simulink model "Lcontainer_simNN"  (R2018b)
settings: Solver=FixedStepAuto  StartTime=0.0  StopTime=600  FixedStep=0.1  RelTol=1e-3
libraries: neural x88, simulink x1
(part 2 of 4)

== system Lcontainer_simNN/LContainer Controller/Layer 2/Delays 1 ==
  "p{2}" : Inport  PortDimensions=10
      mask Display: e = 0.06;c1 = [120 230 180]/255;c2 = ([120 230 180]+0)/(256+128);c3 = ([120 230 180]+128)/(256+128);patch([0 1 1 0],[0 0 1 1],c1);patch([0 1 1 1-e 1-e 0+e],[0 0 1 1-e 0+e 0+e],c2);patch([0 0 1 1-e 0+e 0+e],[0 1 1 1-e 1-e 0+e],c3);plot([0 1 1 0 0],[0 0 1 1 0]);
  mux : Mux  Inputs=1
      mask Display: e = 0.06;c1 = [120 150 230]/255;c2 = ([120 150 230]+0)/383;c3 = ([120 150 230]+128)/383;patch([0 1 1 0],[0 0 1 1],c1);patch([0 1 1 1-e 1-e 0+e],[0 0 1 1-e 0+e 0+e],c2);patch([0 0 1 1-e 0+e 0+e],[0 1 1 1-e 1-e 0+e],c3);plot([0 1 1 0 0],[0 0 1 1 0]);disp('Mux')
  "pd{2,1}" : Outport
      mask Display: e = 0.06;c1 = [120 230 180]/255;c2 = ([120 230 180]+0)/(256+128);c3 = ([120 230 180]+128)/(256+128);patch([0 1 1 0],[0 0 1 1],c1);patch([0 1 1 1-e 1-e 0+e],[0 0 1 1-e 0+e 0+e],c2);patch([0 0 1 1-e 0+e 0+e],[0 1 1 1-e 1-e 0+e],c3);plot([0 1 1 0 0],[0 0 1 1 0]);
  wires:
  mux/1 -> "pd{2,1}"/1
  "p{2}"/1 -> mux/1

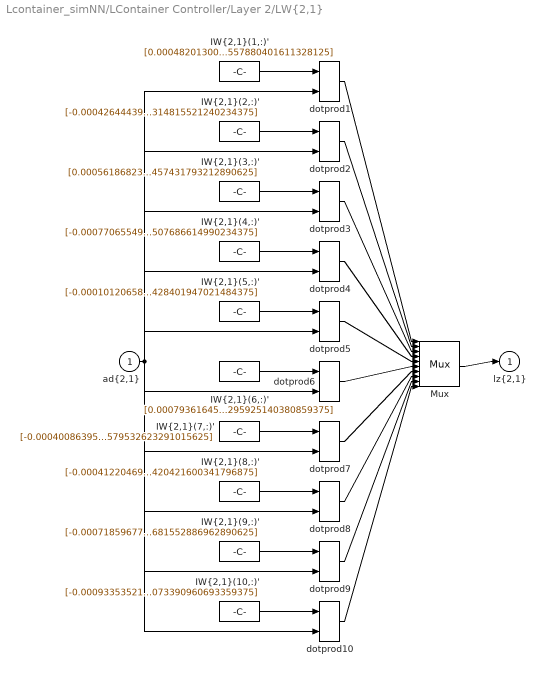
== system Lcontainer_simNN/LContainer Controller/Layer 2/LW{2,1} ==
  "ad{2,1}" : Inport  PortDimensions=10
      mask Display: e = 0.06;c1 = [120 230 180]/255;c2 = ([120 230 180]+0)/(256+128);c3 = ([120 230 180]+128)/(256+128);patch([0 1 1 0],[0 0 1 1],c1);patch([0 1 1 1-e 1-e 0+e],[0 0 1 1-e 0+e 0+e],c2);patch([0 0 1 1-e 0+e 0+e],[0 1 1 1-e 1-e 0+e],c3);plot([0 1 1 0 0],[0 0 1 1 0]);
  "IW{2,1}(1,:)'" : Constant  Value=[0.0004820130050322240893023728602884148131124675273895263671875;-0.14897274999759291258527582613169215619564056396484375;0.0087908951607520609272672373890600283630192279815673828125;-0.053122726519414069368263398018825682811439037322998046875;0.0002402089536153212585845029281017559696920216083526611328125;0.00659270133509061440069132231656112708151340484619140625;0.047066903764155669509516854986941325478255748748779296875;-0.00070479248297768896762416357404390510055236518383026123046875;-0.0302802175473580355291591814648199942894279956817626953125;0.0166965879907191756814643923689800431020557880401611328125]
      mask Display: e = 0.06;c1 = [120 150 230]/255;c2 = ([120 150 230]+0)/383;c3 = ([120 150 230]+128)/383;patch([0 1 1 0],[0 0 1 1],c1);patch([0 1 1 1-e 1-e 0+e],[0 0 1 1-e 0+e 0+e],c2);patch([0 0 1 1-e 0+e 0+e],[0 1 1 1-e 1-e 0+e],c3);plot([0 1 1 0 0],[0 0 1 1 0]);disp('weights');
  "IW{2,1}(10,:)'" : Constant  Value=[-0.000933535212733850269274660238494334407732822000980377197265625;-0.000772387208203969177940095836021328068454749882221221923828125;0.000783528929132344871023863053238756037899293005466461181640625;0.000744496740820047540887482995231039240024983882904052734375;-0.000748280223311167231280138789628608719795010983943939208984375;-0.000336708204216668006113211131236084838747046887874603271484375;-0.000636414158899125162981158521091629154398106038570404052734375;-0.000932538469281236057951967044488128522061742842197418212890625;0.000166570528255750231576282072154526758822612464427947998046875;0.0001092356001364544275909762571785677209845744073390960693359375]
      mask Display: e = 0.06;c1 = [120 150 230]/255;c2 = ([120 150 230]+0)/383;c3 = ([120 150 230]+128)/383;patch([0 1 1 0],[0 0 1 1],c1);patch([0 1 1 1-e 1-e 0+e],[0 0 1 1-e 0+e 0+e],c2);patch([0 0 1 1-e 0+e 0+e],[0 1 1 1-e 1-e 0+e],c3);plot([0 1 1 0 0],[0 0 1 1 0]);disp('weights');
  "IW{2,1}(2,:)'" : Constant  Value=[-0.0004264443902295060964159623129177134615019895136356353759765625;-0.000560105703268952924943346882713512968621216714382171630859375;0.000377584095749465358492213962193773113540373742580413818359375;-0.000700634792845798346459795791218994054361246526241302490234375;0.0004874063537030847402531374967793453834019601345062255859375;-9.7285835613794088990412267659024792010313831269741058349609375e-05;0.000749616668439126465108002239645657027722336351871490478515625;0.00084023165745046525694494921054911173996515572071075439453125;-0.000916171932540294788570311990127947865403257310390472412109375;0.000118539205010998924781639995984505731030367314815521240234375]
      mask Display: e = 0.06;c1 = [120 150 230]/255;c2 = ([120 150 230]+0)/383;c3 = ([120 150 230]+128)/383;patch([0 1 1 0],[0 0 1 1],c1);patch([0 1 1 1-e 1-e 0+e],[0 0 1 1-e 0+e 0+e],c2);patch([0 0 1 1-e 0+e 0+e],[0 1 1 1-e 1-e 0+e],c3);plot([0 1 1 0 0],[0 0 1 1 0]);disp('weights');
  "IW{2,1}(3,:)'" : Constant  Value=[0.000561868235751858554304083437358485753065906465053558349609375;-0.0004553795308148002145276489471825698274187743663787841796875;-0.00016668990031184395951384391576510779486852698028087615966796875;0.000597047158527498384068821213332967090536840260028839111328125;-0.0002934852706778429457488976961343496441259048879146575927734375;0.00015225641794986368338267468391933334714849479496479034423828125;-0.0002772254366225171428629592274006654406548477709293365478515625;0.0003822805927828255173096805297205946772010065615177154541015625;-0.000492935117287975348328299407540953325224108994007110595703125;-0.000934933027334356446004515195369322100304998457431793212890625]
      mask Display: e = 0.06;c1 = [120 150 230]/255;c2 = ([120 150 230]+0)/383;c3 = ([120 150 230]+128)/383;patch([0 1 1 0],[0 0 1 1],c1);patch([0 1 1 1-e 1-e 0+e],[0 0 1 1-e 0+e 0+e],c2);patch([0 0 1 1-e 0+e 0+e],[0 1 1 1-e 1-e 0+e],c3);plot([0 1 1 0 0],[0 0 1 1 0]);disp('weights');
  "IW{2,1}(4,:)'" : Constant  Value=[-0.0007706554936704437981653814659921408747322857379913330078125;0.005736968078448979359296178159866030910052359104156494140625;-0.0215993275616708467479210042938575497828423976898193359375;0.0275851081881576011556322924889173009432852268218994140625;-0.0004468698480519939383003025223928261766559444367885589599609375;-0.0032100621946929267826187359702316825860179960727691650390625;-0.0148528526677068895001099235742003656923770904541015625;-0.00084295935895107947620485955297908731154166162014007568359375;0.0162611889792566959023201178524686838500201702117919921875;-0.03252290811202539211333117918911739252507686614990234375]
      mask Display: e = 0.06;c1 = [120 150 230]/255;c2 = ([120 150 230]+0)/383;c3 = ([120 150 230]+128)/383;patch([0 1 1 0],[0 0 1 1],c1);patch([0 1 1 1-e 1-e 0+e],[0 0 1 1-e 0+e 0+e],c2);patch([0 0 1 1-e 0+e 0+e],[0 1 1 1-e 1-e 0+e],c3);plot([0 1 1 0 0],[0 0 1 1 0]);disp('weights');
  "IW{2,1}(5,:)'" : Constant  Value=[-0.000101206583531268193309506087107507710243226028978824615478515625;-0.000867505466564442322997818823893112494261004030704498291015625;6.972171281489726916112681376347381956293247640132904052734375e-05;-0.0006499836952546214803583257690888785873539745807647705078125;0.000768931164791470550014251816861587940366007387638092041015625;-0.00051077340179170381377626863894647613051347434520721435546875;0.0002396027776789714049988921917844209019676782190799713134765625;0.0004961867667277962933025658998076323769055306911468505859375;7.5421709981156692215002734780426862926105968654155731201171875e-05;-0.0005186449873913457318808095664053325890563428401947021484375]
      mask Display: e = 0.06;c1 = [120 150 230]/255;c2 = ([120 150 230]+0)/383;c3 = ([120 150 230]+128)/383;patch([0 1 1 0],[0 0 1 1],c1);patch([0 1 1 1-e 1-e 0+e],[0 0 1 1-e 0+e 0+e],c2);patch([0 0 1 1-e 0+e 0+e],[0 1 1 1-e 1-e 0+e],c3);plot([0 1 1 0 0],[0 0 1 1 0]);disp('weights');
  "IW{2,1}(6,:)'" : Constant  Value=[0.000793616452609966350865977613437962645548395812511444091796875;0.0072189631106161604445770052507214131765067577362060546875;-0.025168099441065662491556764734923490323126316070556640625;0.03499676826161253473390644330720533616840839385986328125;-0.00013966872952280381145299947842630672312225215137004852294921875;-0.002944584517023267171420553012239906820468604564666748046875;-0.0201810876198396278724533914328276296146214008331298828125;0.000493104595042109512641193003190664967405609786510467529296875;0.0192394162008955559028944293231688789092004299163818359375;-0.040115708372885826304976575329419574700295925140380859375]
      mask Display: e = 0.06;c1 = [120 150 230]/255;c2 = ([120 150 230]+0)/383;c3 = ([120 150 230]+128)/383;patch([0 1 1 0],[0 0 1 1],c1);patch([0 1 1 1-e 1-e 0+e],[0 0 1 1-e 0+e 0+e],c2);patch([0 0 1 1-e 0+e 0+e],[0 1 1 1-e 1-e 0+e],c3);plot([0 1 1 0 0],[0 0 1 1 0]);disp('weights');
  "IW{2,1}(7,:)'" : Constant  Value=[-0.000400863950280058961399276551418324743281118571758270263671875;-0.0225465071540020926821323854483125614933669567108154296875;-0.0280520076515327794475229694626250420697033405303955078125;-0.00942244816999010005587056326703532249666750431060791015625;0.000902860424200245472066417296019835703191347420215606689453125;0.001138975060225336406738438910224431310780346393585205078125;-0.041810146757115640436808234881027601659297943115234375;0.000821642012028902537189301025222221142030321061611175537109375;-0.004447628372272441517332186577959873829968273639678955078125;-0.0285545253020185775538752892543925554491579532623291015625]
      mask Display: e = 0.06;c1 = [120 150 230]/255;c2 = ([120 150 230]+0)/383;c3 = ([120 150 230]+128)/383;patch([0 1 1 0],[0 0 1 1],c1);patch([0 1 1 1-e 1-e 0+e],[0 0 1 1-e 0+e 0+e],c2);patch([0 0 1 1-e 0+e 0+e],[0 1 1 1-e 1-e 0+e],c3);plot([0 1 1 0 0],[0 0 1 1 0]);disp('weights');
  "IW{2,1}(8,:)'" : Constant  Value=[-0.0004122046906352632247329259573831450325087644159793853759765625;-0.50634105157552655729347179658361710608005523681640625;-1.8097291749770356705795393281732685863971710205078125;-0.05223922011666985720790279401626321487128734588623046875;0.000317452984005011664379869440466563901281915605068206787109375;0.00478766364779581975186228959273648797534406185150146484375;-1.1621848213912837621819562627933919429779052734375;0.0004108452670455737111392113813934656718629412353038787841796875;-0.0302623349342728935329471795512290555052459239959716796875;-0.2779400021529727649038932213443331420421600341796875]
      mask Display: e = 0.06;c1 = [120 150 230]/255;c2 = ([120 150 230]+0)/383;c3 = ([120 150 230]+128)/383;patch([0 1 1 0],[0 0 1 1],c1);patch([0 1 1 1-e 1-e 0+e],[0 0 1 1-e 0+e 0+e],c2);patch([0 0 1 1-e 0+e 0+e],[0 1 1 1-e 1-e 0+e],c3);plot([0 1 1 0 0],[0 0 1 1 0]);disp('weights');
  "IW{2,1}(9,:)'" : Constant  Value=[-0.000718596778329273484613171074641968516516499221324920654296875;0.1351387556832968350750689978667651303112506866455078125;-0.069675559698190669966066934648551978170871734619140625;-0.038467952192683417533825007694758824072778224945068359375;0.00023637001640757784003132879746544858790002763271331787109375;0.004472859878445143051728383198906158213503658771514892578125;0.0194364277021570053261001476130331866443157196044921875;-0.00072977980434176729744588651982439841958694159984588623046875;-0.0222208908663231972935303559779640636406838893890380859375;-0.424243744226951324804986143135465681552886962890625]
      mask Display: e = 0.06;c1 = [120 150 230]/255;c2 = ([120 150 230]+0)/383;c3 = ([120 150 230]+128)/383;patch([0 1 1 0],[0 0 1 1],c1);patch([0 1 1 1-e 1-e 0+e],[0 0 1 1-e 0+e 0+e],c2);patch([0 0 1 1-e 0+e 0+e],[0 1 1 1-e 1-e 0+e],c3);plot([0 1 1 0 0],[0 0 1 1 0]);disp('weights');
  Mux : Mux  Inputs=10
      mask Display: e = 0.06;c1 = [120 150 230]/255;c2 = ([120 150 230]+0)/383;c3 = ([120 150 230]+128)/383;patch([0 1 1 0],[0 0 1 1],c1);patch([0 1 1 1-e 1-e 0+e],[0 0 1 1-e 0+e 0+e],c2);patch([0 0 1 1-e 0+e 0+e],[0 1 1 1-e 1-e 0+e],c3);plot([0 1 1 0 0],[0 0 1 1 0]);disp('Mux');
  dotprod{1..10} (10 alike) : neural/Weight Functions/dotprod
  "lz{2,1}" : Outport
      mask Display: e = 0.06;c1 = [120 230 180]/255;c2 = ([120 230 180]+0)/(256+128);c3 = ([120 230 180]+128)/(256+128);patch([0 1 1 0],[0 0 1 1],c1);patch([0 1 1 1-e 1-e 0+e],[0 0 1 1-e 0+e 0+e],c2);patch([0 0 1 1-e 0+e 0+e],[0 1 1 1-e 1-e 0+e],c3);plot([0 1 1 0 0],[0 0 1 1 0]);
  wires:
  Mux/1 -> "lz{2,1}"/1
  dotprod10/1 -> Mux/10
  "IW{2,1}(10,:)'"/1 -> dotprod10/1
  dotprod9/1 -> Mux/9
  "IW{2,1}(9,:)'"/1 -> dotprod9/1
  dotprod8/1 -> Mux/8
  "IW{2,1}(8,:)'"/1 -> dotprod8/1
  dotprod7/1 -> Mux/7
  "IW{2,1}(7,:)'"/1 -> dotprod7/1
  dotprod6/1 -> Mux/6
  "IW{2,1}(6,:)'"/1 -> dotprod6/1
  dotprod5/1 -> Mux/5
  "IW{2,1}(5,:)'"/1 -> dotprod5/1
  dotprod4/1 -> Mux/4
  "IW{2,1}(4,:)'"/1 -> dotprod4/1
  dotprod3/1 -> Mux/3
  "IW{2,1}(3,:)'"/1 -> dotprod3/1
  dotprod2/1 -> Mux/2
  "IW{2,1}(2,:)'"/1 -> dotprod2/1
  dotprod1/1 -> Mux/1
  "ad{2,1}"/1 -> dotprod10/2, dotprod9/2, dotprod8/2, dotprod7/2, dotprod6/2, dotprod5/2, dotprod4/2, dotprod3/2, dotprod2/2, dotprod1/2
  "IW{2,1}(1,:)'"/1 -> dotprod1/1

== system Lcontainer_simNN/LContainer Controller/Layer 3/Delays 1 ==
  "p{3}" : Inport  PortDimensions=10
      mask Display: e = 0.06;c1 = [120 230 180]/255;c2 = ([120 230 180]+0)/(256+128);c3 = ([120 230 180]+128)/(256+128);patch([0 1 1 0],[0 0 1 1],c1);patch([0 1 1 1-e 1-e 0+e],[0 0 1 1-e 0+e 0+e],c2);patch([0 0 1 1-e 0+e 0+e],[0 1 1 1-e 1-e 0+e],c3);plot([0 1 1 0 0],[0 0 1 1 0]);
  mux : Mux  Inputs=1
      mask Display: e = 0.06;c1 = [120 150 230]/255;c2 = ([120 150 230]+0)/383;c3 = ([120 150 230]+128)/383;patch([0 1 1 0],[0 0 1 1],c1);patch([0 1 1 1-e 1-e 0+e],[0 0 1 1-e 0+e 0+e],c2);patch([0 0 1 1-e 0+e 0+e],[0 1 1 1-e 1-e 0+e],c3);plot([0 1 1 0 0],[0 0 1 1 0]);disp('Mux')
  "pd{3,2}" : Outport
      mask Display: e = 0.06;c1 = [120 230 180]/255;c2 = ([120 230 180]+0)/(256+128);c3 = ([120 230 180]+128)/(256+128);patch([0 1 1 0],[0 0 1 1],c1);patch([0 1 1 1-e 1-e 0+e],[0 0 1 1-e 0+e 0+e],c2);patch([0 0 1 1-e 0+e 0+e],[0 1 1 1-e 1-e 0+e],c3);plot([0 1 1 0 0],[0 0 1 1 0]);
  wires:
  mux/1 -> "pd{3,2}"/1
  "p{3}"/1 -> mux/1

== system Lcontainer_simNN/LContainer Controller/Layer 3/LW{3,2} ==
  "ad{3,2}" : Inport  PortDimensions=10
      mask Display: e = 0.06;c1 = [120 230 180]/255;c2 = ([120 230 180]+0)/(256+128);c3 = ([120 230 180]+128)/(256+128);patch([0 1 1 0],[0 0 1 1],c1);patch([0 1 1 1-e 1-e 0+e],[0 0 1 1-e 0+e 0+e],c2);patch([0 0 1 1-e 0+e 0+e],[0 1 1 1-e 1-e 0+e],c3);plot([0 1 1 0 0],[0 0 1 1 0]);
  "IW{3,2}(1,:)'" : Constant  Value=[-0.272649380870168211998816332197748124599456787109375;0.00013227176168331794786463262436626564522157423198223114013671875;-0.00057629457199402677781974180248880657018162310123443603515625;-0.00594714213795307679311097359686755225993692874908447265625;0.0004735837959567169006859510549389824518584646284580230712890625;-0.037568305788482865559263501609166269190609455108642578125;0.00724237752689754592239079755700004170648753643035888671875;-2.15262859222610369869244095752947032451629638671875;0.058953518285207950899717843640246428549289703369140625;-0.00050529459321236648051967055295108366408385336399078369140625]
      mask Display: e = 0.06;c1 = [120 150 230]/255;c2 = ([120 150 230]+0)/383;c3 = ([120 150 230]+128)/383;patch([0 1 1 0],[0 0 1 1],c1);patch([0 1 1 1-e 1-e 0+e],[0 0 1 1-e 0+e 0+e],c2);patch([0 0 1 1-e 0+e 0+e],[0 1 1 1-e 1-e 0+e],c3);plot([0 1 1 0 0],[0 0 1 1 0]);disp('weights');
  Mux : Mux  Inputs=1
      mask Display: e = 0.06;c1 = [120 150 230]/255;c2 = ([120 150 230]+0)/383;c3 = ([120 150 230]+128)/383;patch([0 1 1 0],[0 0 1 1],c1);patch([0 1 1 1-e 1-e 0+e],[0 0 1 1-e 0+e 0+e],c2);patch([0 0 1 1-e 0+e 0+e],[0 1 1 1-e 1-e 0+e],c3);plot([0 1 1 0 0],[0 0 1 1 0]);disp('Mux');
  dotprod1 : neural/Weight Functions/dotprod
  "lz{3,2}" : Outport
      mask Display: e = 0.06;c1 = [120 230 180]/255;c2 = ([120 230 180]+0)/(256+128);c3 = ([120 230 180]+128)/(256+128);patch([0 1 1 0],[0 0 1 1],c1);patch([0 1 1 1-e 1-e 0+e],[0 0 1 1-e 0+e 0+e],c2);patch([0 0 1 1-e 0+e 0+e],[0 1 1 1-e 1-e 0+e],c3);plot([0 1 1 0 0],[0 0 1 1 0]);
  wires:
  Mux/1 -> "lz{3,2}"/1
  dotprod1/1 -> Mux/1
  "ad{3,2}"/1 -> dotprod1/2
  "IW{3,2}(1,:)'"/1 -> dotprod1/1

== system Lcontainer_simNN/LContainer Plant/Layer 1/Delays 1 ==
  "p{1}" : Inport  PortDimensions=10
      mask Display: e = 0.06;c1 = [120 230 180]/255;c2 = ([120 230 180]+0)/(256+128);c3 = ([120 230 180]+128)/(256+128);patch([0 1 1 0],[0 0 1 1],c1);patch([0 1 1 1-e 1-e 0+e],[0 0 1 1-e 0+e 0+e],c2);patch([0 0 1 1-e 0+e 0+e],[0 1 1 1-e 1-e 0+e],c3);plot([0 1 1 0 0],[0 0 1 1 0]);
  mux : Mux  Inputs=1
      mask Display: e = 0.06;c1 = [120 150 230]/255;c2 = ([120 150 230]+0)/383;c3 = ([120 150 230]+128)/383;patch([0 1 1 0],[0 0 1 1],c1);patch([0 1 1 1-e 1-e 0+e],[0 0 1 1-e 0+e 0+e],c2);patch([0 0 1 1-e 0+e 0+e],[0 1 1 1-e 1-e 0+e],c3);plot([0 1 1 0 0],[0 0 1 1 0]);disp('Mux')
  "pd{1,1}" : Outport
      mask Display: e = 0.06;c1 = [120 230 180]/255;c2 = ([120 230 180]+0)/(256+128);c3 = ([120 230 180]+128)/(256+128);patch([0 1 1 0],[0 0 1 1],c1);patch([0 1 1 1-e 1-e 0+e],[0 0 1 1-e 0+e 0+e],c2);patch([0 0 1 1-e 0+e 0+e],[0 1 1 1-e 1-e 0+e],c3);plot([0 1 1 0 0],[0 0 1 1 0]);
  wires:
  mux/1 -> "pd{1,1}"/1
  "p{1}"/1 -> mux/1

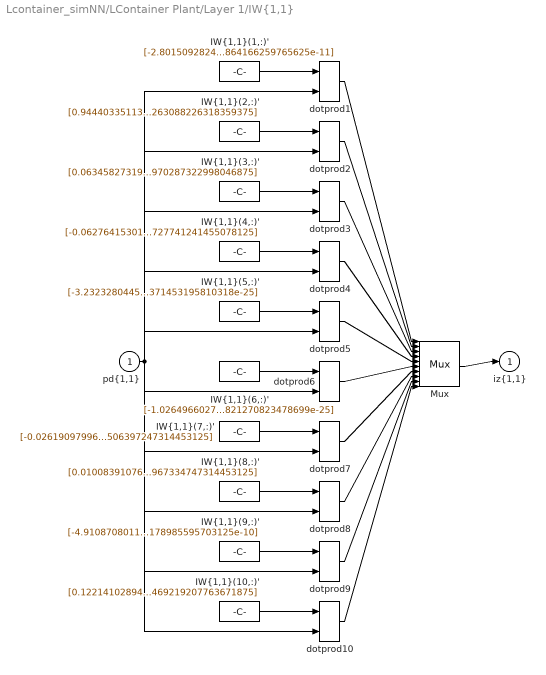
== system Lcontainer_simNN/LContainer Plant/Layer 1/IW{1,1} ==
  "pd{1,1}" : Inport  PortDimensions=10
      mask Display: e = 0.06;c1 = [120 230 180]/255;c2 = ([120 230 180]+0)/(256+128);c3 = ([120 230 180]+128)/(256+128);patch([0 1 1 0],[0 0 1 1],c1);patch([0 1 1 1-e 1-e 0+e],[0 0 1 1-e 0+e 0+e],c2);patch([0 0 1 1-e 0+e 0+e],[0 1 1 1-e 1-e 0+e],c3);plot([0 1 1 0 0],[0 0 1 1 0]);
  "IW{1,1}(1,:)'" : Constant  Value=[-2.801509282442014055289999211492517339205932103141094557940959930419921875e-09;6.48709663420110913726937300883526767159015236074992571957409381866455078125e-11;-1.38806045741189341650107961675240076889793761072411371060297824442386627197265625e-12;-6.949262728077942046686543068993724414639245878788642585277557373046875e-10;4.9583045758239326267706093454186444535736200123210437595844268798828125e-09;7.20807982755057124969425602884896237096575000169451641340856440365314483642578125e-13;1.47915336545584584323170595539991166640116093677903563730069436132907867431640625e-12;1.368467688852383455193129604555463631654528555703365100271184928715229034423828125e-13;-2.4782259643928960868026404257559685943845817490682748029939830303192138671875e-11;-2.17656041339324496223947102679151612870944720867782962159253656864166259765625e-11]
      mask Display: e = 0.06;c1 = [120 150 230]/255;c2 = ([120 150 230]+0)/383;c3 = ([120 150 230]+128)/383;patch([0 1 1 0],[0 0 1 1],c1);patch([0 1 1 1-e 1-e 0+e],[0 0 1 1-e 0+e 0+e],c2);patch([0 0 1 1-e 0+e 0+e],[0 1 1 1-e 1-e 0+e],c3);plot([0 1 1 0 0],[0 0 1 1 0]);disp('Weights');
  "IW{1,1}(10,:)'" : Constant  Value=[0.1221410289429804285621372628156677819788455963134765625;-0.06221579091204963718464426847276627086102962493896484375;0.00077577425811804832760099071009562976541928946971893310546875;0.0057878098276135346578197271583121619187295436859130859375;-0.29336456194867477353938056694460101425647735595703125;-0.00153674477675105609734973466373730843770317733287811279296875;-0.01024849367676159382634093475417103036306798458099365234375;0.07417790242423320801190556039728107862174510955810546875;-0.1474125279109223252138605175787233747541904449462890625;0.67016334654499143397288207779638469219207763671875]
      mask Display: e = 0.06;c1 = [120 150 230]/255;c2 = ([120 150 230]+0)/383;c3 = ([120 150 230]+128)/383;patch([0 1 1 0],[0 0 1 1],c1);patch([0 1 1 1-e 1-e 0+e],[0 0 1 1-e 0+e 0+e],c2);patch([0 0 1 1-e 0+e 0+e],[0 1 1 1-e 1-e 0+e],c3);plot([0 1 1 0 0],[0 0 1 1 0]);disp('Weights');
  "IW{1,1}(2,:)'" : Constant  Value=[0.94440335113838036473765669143176637589931488037109375;-0.1629366186686034001507294988186913542449474334716796875;0.0014086521436272440334358524438584936433471739292144775390625;0.0011875416120418805752956270538334138109348714351654052734375;-0.0095127288471239003497803565778667689301073551177978515625;-0.030355092939376430993814182102141785435378551483154296875;-0.027077648132769714661716164982863119803369045257568359375;-0.0214545100883952628845197097007257980294525623321533203125;0.0221409157462193577348141815264170872978866100311279296875;-0.0799528339554468059358072196118882857263088226318359375]
      mask Display: e = 0.06;c1 = [120 150 230]/255;c2 = ([120 150 230]+0)/383;c3 = ([120 150 230]+128)/383;patch([0 1 1 0],[0 0 1 1],c1);patch([0 1 1 1-e 1-e 0+e],[0 0 1 1-e 0+e 0+e],c2);patch([0 0 1 1-e 0+e 0+e],[0 1 1 1-e 1-e 0+e],c3);plot([0 1 1 0 0],[0 0 1 1 0]);disp('Weights');
  "IW{1,1}(3,:)'" : Constant  Value=[0.06345827319009154920959048240547417663037776947021484375;-0.002284892575671929569602891518798060133121907711029052734375;-3.8590476702913398461027016939084433033713139593601226806640625e-05;-0.0110663773782371521736678232628037221729755401611328125;-0.0908700265878994162260795519614475779235363006591796875;0.000526541045885379967346484608725631915149278938770294189453125;-0.0003614651660661234136746877698698199310456402599811553955078125;7.84278586458189426282305856119592135655693709850311279296875e-05;-0.0134962408454888278808159185473414254374802112579345703125;0.149807902282869942478527036655577830970287322998046875]
      mask Display: e = 0.06;c1 = [120 150 230]/255;c2 = ([120 150 230]+0)/383;c3 = ([120 150 230]+128)/383;patch([0 1 1 0],[0 0 1 1],c1);patch([0 1 1 1-e 1-e 0+e],[0 0 1 1-e 0+e 0+e],c2);patch([0 0 1 1-e 0+e 0+e],[0 1 1 1-e 1-e 0+e],c3);plot([0 1 1 0 0],[0 0 1 1 0]);disp('Weights');
  "IW{1,1}(4,:)'" : Constant  Value=[-0.06276415301526915013763385786660364829003810882568359375;0.299133911149455367084470935878925956785678863525390625;-0.00136204698319966643373091219615389491082169115543365478515625;0.0380217836961479760393700644272030331194400787353515625;-0.32048901761800208110031462638289667665958404541015625;0.00785310746361885143873582393325705197639763355255126953125;0.0759200265843099908469326919657760299742221832275390625;-0.21764633419310241979616193930269218981266021728515625;0.01506368619694353240545670047367821098305284976959228515625;0.00498490442438284837856077302831181441433727741241455078125]
      mask Display: e = 0.06;c1 = [120 150 230]/255;c2 = ([120 150 230]+0)/383;c3 = ([120 150 230]+128)/383;patch([0 1 1 0],[0 0 1 1],c1);patch([0 1 1 1-e 1-e 0+e],[0 0 1 1-e 0+e 0+e],c2);patch([0 0 1 1-e 0+e 0+e],[0 1 1 1-e 1-e 0+e],c3);plot([0 1 1 0 0],[0 0 1 1 0]);disp('Weights');
  "IW{1,1}(5,:)'" : Constant  Value=[-3.232328044521501967189195073260012196184779564093179990637908470269695770937801171385217458009719849e-24;1.27219627644899788443117073026932678970995136194323539365026960528629734747951829376688692718744278e-24;-2.304586043009832518419089320741620377711305370506937496231022479385719403666143989539705216884613037e-24;-3.65383458475199811491012570879355089482131624352566575712094985731517859939287973247701302170753479e-24;7.841466587439908830490789390900702708149702478533912974227431931604354042875115737842861562967300415e-25;-3.59690334700841611751283031893362553567812437986740933047257286810788334818766998068895190954208374e-24;6.165357822344626074123519954547509568304369779818255337247319736756860641957445068328524939715862274e-25;-3.641944249061509432581116542493658345326055739461618632621637636857109265875465098361019045114517212e-24;-3.353455415433941917570106955630704025672682003188821480519606142278038474202617180708330124616622925e-24;5.61638438383968347577255870017047939309716900375765715826956117498556381173457907607371453195810318e-25]
      mask Display: e = 0.06;c1 = [120 150 230]/255;c2 = ([120 150 230]+0)/383;c3 = ([120 150 230]+128)/383;patch([0 1 1 0],[0 0 1 1],c1);patch([0 1 1 1-e 1-e 0+e],[0 0 1 1-e 0+e 0+e],c2);patch([0 0 1 1-e 0+e 0+e],[0 1 1 1-e 1-e 0+e],c3);plot([0 1 1 0 0],[0 0 1 1 0]);disp('Weights');
  "IW{1,1}(6,:)'" : Constant  Value=[-1.026496602779318694400227172068556650717545644267548449537601734825255535288324182374708470888435841e-25;-1.767200554431897263726751072979481661861387311042597372530084289931479046842355273838620632886886597e-24;1.048387282269173117106175616203935637006982073632968147776087025017238696378285567334387451410293579e-24;-1.996914179418175239613798079100530232733597892032674775672844403543587654681346066354308277368545532e-24;3.724729865716098500094696689779701389908161006250711819853465012729060862328722691927396226674318314e-25;3.367584298875349568394472393583656104771561930333680381613226150275264281219733675243332982063293457e-24;2.847842577594690823339253670797999667900935394680387375414817375304105118161146492639090865850448608e-24;7.027398573851468269303495927700750972016986923806031058583281391841102170303656748728826642036437988e-25;-5.9993835158433249173768534931805326185402475759469404997544781700264532320332477866031695157289505e-25;9.628037386970728061986184227006127764244953076546257034527088119286661327400622667482821270823478699e-25]
      mask Display: e = 0.06;c1 = [120 150 230]/255;c2 = ([120 150 230]+0)/383;c3 = ([120 150 230]+128)/383;patch([0 1 1 0],[0 0 1 1],c1);patch([0 1 1 1-e 1-e 0+e],[0 0 1 1-e 0+e 0+e],c2);patch([0 0 1 1-e 0+e 0+e],[0 1 1 1-e 1-e 0+e],c3);plot([0 1 1 0 0],[0 0 1 1 0]);disp('Weights');
  "IW{1,1}(7,:)'" : Constant  Value=[-0.0261909799619371892742680785204356652684509754180908203125;0.0003437492496853357393238326267237425781786441802978515625;-1.036955602107424352122111432805695585557259619235992431640625e-05;-0.00932767157300501241479206981921379338018596172332763671875;-0.01229205498181146390124229839102554251439869403839111328125;0.00020759065297099415212979389711023259224020875990390777587890625;1.08964068133936734070373042460033730094437487423419952392578125e-05;-2.561171802817354911131764172438352034077979624271392822265625e-05;-0.000287688264983173235499191999764434513053856790065765380859375;-0.00043040854605869084854863348965636760112829506397247314453125]
      mask Display: e = 0.06;c1 = [120 150 230]/255;c2 = ([120 150 230]+0)/383;c3 = ([120 150 230]+128)/383;patch([0 1 1 0],[0 0 1 1],c1);patch([0 1 1 1-e 1-e 0+e],[0 0 1 1-e 0+e 0+e],c2);patch([0 0 1 1-e 0+e 0+e],[0 1 1 1-e 1-e 0+e],c3);plot([0 1 1 0 0],[0 0 1 1 0]);disp('Weights');
  "IW{1,1}(8,:)'" : Constant  Value=[0.0100839107691757003115728963393848971463739871978759765625;-0.003764502474562787803780139483933453448116779327392578125;0.000104505260114816042084362468500557952211238443851470947265625;-0.011361695267675019083153387100537656806409358978271484375;-0.05599864890587578913905275612705736421048641204833984375;-0.00018576636026189908526724814397113050290499813854694366455078125;8.610962378234558582158764128422490102821029722690582275390625e-06;0.00017937370587163632067000118563981914121541194617748260498046875;-0.11442264161428827851096912127104587852954864501953125;0.79119009598240996883333764344570226967334747314453125]
      mask Display: e = 0.06;c1 = [120 150 230]/255;c2 = ([120 150 230]+0)/383;c3 = ([120 150 230]+128)/383;patch([0 1 1 0],[0 0 1 1],c1);patch([0 1 1 1-e 1-e 0+e],[0 0 1 1-e 0+e 0+e],c2);patch([0 0 1 1-e 0+e 0+e],[0 1 1 1-e 1-e 0+e],c3);plot([0 1 1 0 0],[0 0 1 1 0]);disp('Weights');
  "IW{1,1}(9,:)'" : Constant  Value=[-4.91087080115513649427431172415914328865937932278029620647430419921875e-09;-3.0590489359197964948747691596244477167665376526883846963755786418914794921875e-11;-2.227568969543201563024170237666836858099472795657902679522521793842315673828125e-13;-2.222671677422157718647604926050990840902255030187006923370063304901123046875e-10;-7.553563145234592475399415208427655009371104455340173444710671901702880859375e-11;9.43329368888154045226968570842830674738621610231348313391208648681640625e-12;-3.992753603625621062081869849271281909010300470441734432824887335300445556640625e-12;7.5776284623655886182437955066170463922121947053511803460423834621906280517578125e-13;-3.056807526493178000986899905716716319137304935793508775532245635986328125e-10;-1.1572160074794368434413739157908267325691742399840222788043320178985595703125e-10]
      mask Display: e = 0.06;c1 = [120 150 230]/255;c2 = ([120 150 230]+0)/383;c3 = ([120 150 230]+128)/383;patch([0 1 1 0],[0 0 1 1],c1);patch([0 1 1 1-e 1-e 0+e],[0 0 1 1-e 0+e 0+e],c2);patch([0 0 1 1-e 0+e 0+e],[0 1 1 1-e 1-e 0+e],c3);plot([0 1 1 0 0],[0 0 1 1 0]);disp('Weights');
  Mux : Mux  Inputs=10
      mask Display: e = 0.06;c1 = [120 150 230]/255;c2 = ([120 150 230]+0)/383;c3 = ([120 150 230]+128)/383;patch([0 1 1 0],[0 0 1 1],c1);patch([0 1 1 1-e 1-e 0+e],[0 0 1 1-e 0+e 0+e],c2);patch([0 0 1 1-e 0+e 0+e],[0 1 1 1-e 1-e 0+e],c3);plot([0 1 1 0 0],[0 0 1 1 0]);disp('Mux');
  dotprod{1..10} (10 alike) : neural/Weight Functions/dotprod
  "iz{1,1}" : Outport
      mask Display: e = 0.06;c1 = [120 230 180]/255;c2 = ([120 230 180]+0)/(256+128);c3 = ([120 230 180]+128)/(256+128);patch([0 1 1 0],[0 0 1 1],c1);patch([0 1 1 1-e 1-e 0+e],[0 0 1 1-e 0+e 0+e],c2);patch([0 0 1 1-e 0+e 0+e],[0 1 1 1-e 1-e 0+e],c3);plot([0 1 1 0 0],[0 0 1 1 0]);
  wires:
  Mux/1 -> "iz{1,1}"/1
  dotprod10/1 -> Mux/10
  "IW{1,1}(10,:)'"/1 -> dotprod10/1
  dotprod9/1 -> Mux/9
  "IW{1,1}(9,:)'"/1 -> dotprod9/1
  dotprod8/1 -> Mux/8
  "IW{1,1}(8,:)'"/1 -> dotprod8/1
  dotprod7/1 -> Mux/7
  "IW{1,1}(7,:)'"/1 -> dotprod7/1
  dotprod6/1 -> Mux/6
  "IW{1,1}(6,:)'"/1 -> dotprod6/1
  dotprod5/1 -> Mux/5
  "IW{1,1}(5,:)'"/1 -> dotprod5/1
  dotprod4/1 -> Mux/4
  "IW{1,1}(4,:)'"/1 -> dotprod4/1
  dotprod3/1 -> Mux/3
  "IW{1,1}(3,:)'"/1 -> dotprod3/1
  dotprod2/1 -> Mux/2
  "IW{1,1}(2,:)'"/1 -> dotprod2/1
  dotprod1/1 -> Mux/1
  "pd{1,1}"/1 -> dotprod10/2, dotprod9/2, dotprod8/2, dotprod7/2, dotprod6/2, dotprod5/2, dotprod4/2, dotprod3/2, dotprod2/2, dotprod1/2
  "IW{1,1}(1,:)'"/1 -> dotprod1/1

== system Lcontainer_simNN/LContainer Plant/Layer 2/Delays 1 ==
  "p{2}" : Inport  PortDimensions=10
      mask Display: e = 0.06;c1 = [120 230 180]/255;c2 = ([120 230 180]+0)/(256+128);c3 = ([120 230 180]+128)/(256+128);patch([0 1 1 0],[0 0 1 1],c1);patch([0 1 1 1-e 1-e 0+e],[0 0 1 1-e 0+e 0+e],c2);patch([0 0 1 1-e 0+e 0+e],[0 1 1 1-e 1-e 0+e],c3);plot([0 1 1 0 0],[0 0 1 1 0]);
  mux : Mux  Inputs=1
      mask Display: e = 0.06;c1 = [120 150 230]/255;c2 = ([120 150 230]+0)/383;c3 = ([120 150 230]+128)/383;patch([0 1 1 0],[0 0 1 1],c1);patch([0 1 1 1-e 1-e 0+e],[0 0 1 1-e 0+e 0+e],c2);patch([0 0 1 1-e 0+e 0+e],[0 1 1 1-e 1-e 0+e],c3);plot([0 1 1 0 0],[0 0 1 1 0]);disp('Mux')
  "pd{2,1}" : Outport
      mask Display: e = 0.06;c1 = [120 230 180]/255;c2 = ([120 230 180]+0)/(256+128);c3 = ([120 230 180]+128)/(256+128);patch([0 1 1 0],[0 0 1 1],c1);patch([0 1 1 1-e 1-e 0+e],[0 0 1 1-e 0+e 0+e],c2);patch([0 0 1 1-e 0+e 0+e],[0 1 1 1-e 1-e 0+e],c3);plot([0 1 1 0 0],[0 0 1 1 0]);
  wires:
  mux/1 -> "pd{2,1}"/1
  "p{2}"/1 -> mux/1

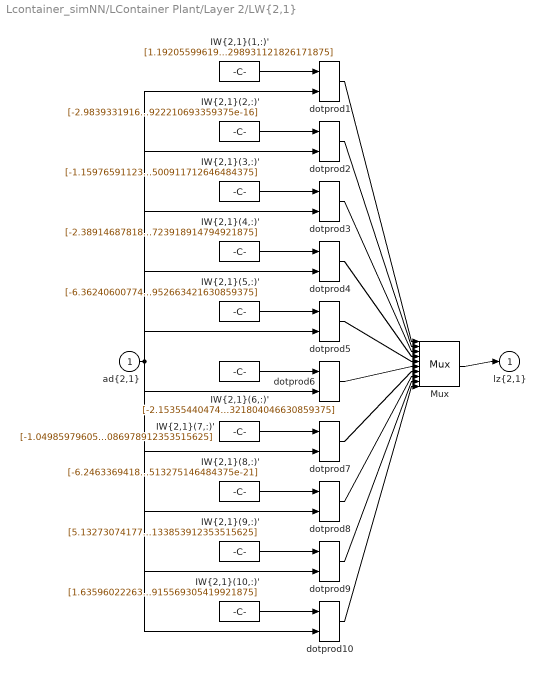
== system Lcontainer_simNN/LContainer Plant/Layer 2/LW{2,1} ==
  "ad{2,1}" : Inport  PortDimensions=10
      mask Display: e = 0.06;c1 = [120 230 180]/255;c2 = ([120 230 180]+0)/(256+128);c3 = ([120 230 180]+128)/(256+128);patch([0 1 1 0],[0 0 1 1],c1);patch([0 1 1 1-e 1-e 0+e],[0 0 1 1-e 0+e 0+e],c2);patch([0 0 1 1-e 0+e 0+e],[0 1 1 1-e 1-e 0+e],c3);plot([0 1 1 0 0],[0 0 1 1 0]);
  "IW{2,1}(1,:)'" : Constant  Value=[1.19205599619928425637544055376050577965685306480736471712589263916015625e-09;0.859783473122643027153344519319944083690643310546875;-0.0232952995570454741980359614217377384193241596221923828125;-0.019153240979415335487612281895053456537425518035888671875;-1.825846003103510989403161386848035542536052237189832903179332045410718232680835626524640247225761414e-24;-2.002145912565504333693414121413473990240941507787062699464222440383712187106368673994438722729682922e-24;-0.002395826527032540211037403565796921611763536930084228515625;0.000546771968617274753583779034471490376745350658893585205078125;-1.953009345362034143028492880786277374749460022940183989703655242919921875e-09;-0.06782547419955346768016823943980853073298931121826171875]
      mask Display: e = 0.06;c1 = [120 150 230]/255;c2 = ([120 150 230]+0)/383;c3 = ([120 150 230]+128)/383;patch([0 1 1 0],[0 0 1 1],c1);patch([0 1 1 1-e 1-e 0+e],[0 0 1 1-e 0+e 0+e],c2);patch([0 0 1 1-e 0+e 0+e],[0 1 1 1-e 1-e 0+e],c3);plot([0 1 1 0 0],[0 0 1 1 0]);disp('weights');
  "IW{2,1}(10,:)'" : Constant  Value=[1.63596022263663484426641497458849994206531164309126324951648712158203125e-09;-0.06858503111573154009672492747995420359075069427490234375;0.024825265048579965576625028234047931618988513946533203125;-0.07256814905749871258411332064497401006519794464111328125;8.771717177242344629328060905286938799894811548117259953516228790067546516873164819116936996579170227e-25;1.890842528295030023215404073031365490773123369053786422164396607619937795696785087784519419074058533e-24;0.0205276887596622277520896915348203037865459918975830078125;0.6834698110443022667226387056871317327022552490234375;-3.70371695649537989037189609207480212038632316762232221662998199462890625e-09;0.5070683938200069018620297356392256915569305419921875]
      mask Display: e = 0.06;c1 = [120 150 230]/255;c2 = ([120 150 230]+0)/383;c3 = ([120 150 230]+128)/383;patch([0 1 1 0],[0 0 1 1],c1);patch([0 1 1 1-e 1-e 0+e],[0 0 1 1-e 0+e 0+e],c2);patch([0 0 1 1-e 0+e 0+e],[0 1 1 1-e 1-e 0+e],c3);plot([0 1 1 0 0],[0 0 1 1 0]);disp('weights');
  "IW{2,1}(2,:)'" : Constant  Value=[-2.983933191664753650225232331897141378024049360347114134839330290560610592365264892578125e-16;-5.549381103871049382208627705545478708265148999612126345937213045544922351837158203125e-16;-4.481730015212207284056274954223401083919657073885434162008323255577124655246734619140625e-16;-3.274415733856125896844625936865109498298729803246465142052556984708644449710845947265625e-16;-2.925097055501374738370434847233118085837935614447137668454811359856904129372878742287866771221160889e-24;-2.992182901698807986741570106278618637195168248877016719304394021640772227677018690883414819836616516e-24;-1.41092943616204682641309453912043857254024012567138190998861091429716907441616058349609375e-16;-5.8057074732073900001506253537644557680556301783314498976551476516760885715484619140625e-16;-5.650214129431145112787162180978964880336692737893000693105705067864619195461273193359375e-16;-2.30482998785585517911639410363769578425638200579184111660424605361185967922210693359375e-16]
      mask Display: e = 0.06;c1 = [120 150 230]/255;c2 = ([120 150 230]+0)/383;c3 = ([120 150 230]+128)/383;patch([0 1 1 0],[0 0 1 1],c1);patch([0 1 1 1-e 1-e 0+e],[0 0 1 1-e 0+e 0+e],c2);patch([0 0 1 1-e 0+e 0+e],[0 1 1 1-e 1-e 0+e],c3);plot([0 1 1 0 0],[0 0 1 1 0]);disp('weights');
  "IW{2,1}(3,:)'" : Constant  Value=[-1.159765911235507771982627898943972455381157260489999316632747650146484375e-09;0.41810556621323746728791093119070865213871002197265625;0.04854057673964669306077013288813759572803974151611328125;-0.06219987416265458646247310525723150931298732757568359375;-2.308130888969874611838483505469665058650466908181076557066053491201057523696249518252443522214889526e-24;1.192040006598243972585233133379346411177907773712728809487686505047022988978966395734460093080997467e-25;-0.0238654034781258898856304284663565340451896190643310546875;0.27572259003480115158168928246595896780490875244140625;-8.3066011083839105814817494770536422665774267670713015832006931304931640625e-10;0.1640934167286230704885241493684588931500911712646484375]
      mask Display: e = 0.06;c1 = [120 150 230]/255;c2 = ([120 150 230]+0)/383;c3 = ([120 150 230]+128)/383;patch([0 1 1 0],[0 0 1 1],c1);patch([0 1 1 1-e 1-e 0+e],[0 0 1 1-e 0+e 0+e],c2);patch([0 0 1 1-e 0+e 0+e],[0 1 1 1-e 1-e 0+e],c3);plot([0 1 1 0 0],[0 0 1 1 0]);disp('weights');
  "IW{2,1}(4,:)'" : Constant  Value=[-2.389146878183538179533425220416910372822627550704055465757846832275390625e-09;0.1571028799736538250630957236353424377739429473876953125;0.035000789761108257180932668006789754144847393035888671875;-0.1012297104985324380788114240203867666423320770263671875;-3.125967434557596407525067421939005067273883086879381809200613704669555800025326774971290433313697577e-27;-1.718410089381724417831967507179645552765880837135342249497508168397516201131303148486040299758315086e-25;-0.0275861972183955757309536949151151929982006549835205078125;-0.2449647270787025654659174733751569874584674835205078125;-1.7175722743397535300090630077632543326604519506872748024761676788330078125e-09;-0.258277851840702232788515857464517466723918914794921875]
      mask Display: e = 0.06;c1 = [120 150 230]/255;c2 = ([120 150 230]+0)/383;c3 = ([120 150 230]+128)/383;patch([0 1 1 0],[0 0 1 1],c1);patch([0 1 1 1-e 1-e 0+e],[0 0 1 1-e 0+e 0+e],c2);patch([0 0 1 1-e 0+e 0+e],[0 1 1 1-e 1-e 0+e],c3);plot([0 1 1 0 0],[0 0 1 1 0]);disp('weights');
  "IW{2,1}(5,:)'" : Constant  Value=[-6.36240600774908972831819464689891152620049297183868475258350372314453125e-09;0.08784451538395289527105802562800818122923374176025390625;0.0778888854190530610654974452700116671621799468994140625;-0.15798995041492125412929681260720826685428619384765625;1.71837655007121259503033687287020860216680196204435722288379203388439253608055423683254048228263855e-24;-2.611016286203771938348552330440559128774908894829158935122512350673895653585532272700220346450805664e-24;-0.0306662956038743945985647343377422657795250415802001953125;0.173324100522433022231183485928340815007686614990234375;-4.23301131317589036458555129213178480629409250468597747385501861572265625e-09;0.200813714629148376555889399242005310952663421630859375]
      mask Display: e = 0.06;c1 = [120 150 230]/255;c2 = ([120 150 230]+0)/383;c3 = ([120 150 230]+128)/383;patch([0 1 1 0],[0 0 1 1],c1);patch([0 1 1 1-e 1-e 0+e],[0 0 1 1-e 0+e 0+e],c2);patch([0 0 1 1-e 0+e 0+e],[0 1 1 1-e 1-e 0+e],c3);plot([0 1 1 0 0],[0 0 1 1 0]);disp('weights');
  "IW{2,1}(6,:)'" : Constant  Value=[-2.15355440474474276533495777541556137624212396985967643558979034423828125e-09;0.11756913123664748666019619349754066206514835357666015625;0.09467565912922364101955707837987574748694896697998046875;0.2173871075974486977155919475990231148898601531982421875;-2.193627617175477446949431586928176145115951719006207065935724323437611138487568496202584356069564819e-24;9.156697097230096239772156423767029498990931682827442369988723799064528341418167656229343265295028687e-25;-0.017534523044202277031189396439003758132457733154296875;-0.0770418601774521538683160315486020408570766448974609375;-1.587264677030336731948463035459483128075675040236092172563076019287109375e-09;-0.028084608300217993315239795037996373139321804046630859375]
      mask Display: e = 0.06;c1 = [120 150 230]/255;c2 = ([120 150 230]+0)/383;c3 = ([120 150 230]+128)/383;patch([0 1 1 0],[0 0 1 1],c1);patch([0 1 1 1-e 1-e 0+e],[0 0 1 1-e 0+e 0+e],c2);patch([0 0 1 1-e 0+e 0+e],[0 1 1 1-e 1-e 0+e],c3);plot([0 1 1 0 0],[0 0 1 1 0]);disp('weights');
  "IW{2,1}(7,:)'" : Constant  Value=[-1.04985979605989152920102753098301195944230812528985552489757537841796875e-08;0.290189826300936426495269415681832469999790191650390625;0.11196067217704101792730142506115953437983989715576171875;-0.18187139211849745468185801655636169016361236572265625;-1.89413985836386170317638850272351490528292454918607953584980306896423662976758350851014256477355957e-24;3.308429472951996360436280118004689843492831666244703632338073366798720381654064226495393086224794388e-25;-0.0228421041888604882397206807809197925962507724761962890625;0.053849327210877560856427948010605177842080593109130859375;-1.2023613697432434633246284695455574631495210269349627196788787841796875e-08;0.239995223940939139684047631817520596086978912353515625]
      mask Display: e = 0.06;c1 = [120 150 230]/255;c2 = ([120 150 230]+0)/383;c3 = ([120 150 230]+128)/383;patch([0 1 1 0],[0 0 1 1],c1);patch([0 1 1 1-e 1-e 0+e],[0 0 1 1-e 0+e 0+e],c2);patch([0 0 1 1-e 0+e 0+e],[0 1 1 1-e 1-e 0+e],c3);plot([0 1 1 0 0],[0 0 1 1 0]);disp('weights');
  "IW{2,1}(8,:)'" : Constant  Value=[-6.246336941884103552009331633563366933978605083498984494670257933135459893492225091904401779174804688e-22;-6.118209702480057750190044547641385185706143708903940168532253895961048328899778425693511962890625e-20;-3.0817079067971096623659228441087988752480355875440159551907626234168446899275295436382293701171875e-20;-5.285070250538343101132739947163877753416697363837277004222810206091054396893014200031757354736328125e-22;2.643668381308280100565792459086614133351635145852596615377212582948321384357370789075503125786781311e-24;1.15871657594034666187772576796443740445192343217831120673811837965688775753392292244825512170791626e-24;2.889744289645617124314059885944833331713212898732063417292485158296456992932377261240617372095584869e-25;-1.96689619001296129044047415961882850404253629524781819414187833405804894937318749725818634033203125e-20;-5.05713832988823791166125172503428194592625212822460689134074218742398443282581865787506103515625e-20;-8.764989521086254731690224871934214675019891863845476732107486750322777879773639142513275146484375e-21]
      mask Display: e = 0.06;c1 = [120 150 230]/255;c2 = ([120 150 230]+0)/383;c3 = ([120 150 230]+128)/383;patch([0 1 1 0],[0 0 1 1],c1);patch([0 1 1 1-e 1-e 0+e],[0 0 1 1-e 0+e 0+e],c2);patch([0 0 1 1-e 0+e 0+e],[0 1 1 1-e 1-e 0+e],c3);plot([0 1 1 0 0],[0 0 1 1 0]);disp('weights');
  "IW{2,1}(9,:)'" : Constant  Value=[5.1327307417752188318460246992287754341788286183145828545093536376953125e-09;0.01951913301069409245602770397454150952398777008056640625;0.055433637241927326277934895415455684997141361236572265625;0.09791259364152964106420284906562301330268383026123046875;-6.326012932940250038371281041983775345382603702682803760972385343722829142976138427911791950464248657e-25;-2.672103696908223499170502996448574659547387081788547362707536873219910100729634905292186886072158813e-24;0.023081397355434886409231154402732499875128269195556640625;0.0267995661430773281230788285256494418717920780181884765625;-3.7741115409921664832198695744593097689545402317889966070652008056640625e-09;-0.307809122913129284970779053764999844133853912353515625]
      mask Display: e = 0.06;c1 = [120 150 230]/255;c2 = ([120 150 230]+0)/383;c3 = ([120 150 230]+128)/383;patch([0 1 1 0],[0 0 1 1],c1);patch([0 1 1 1-e 1-e 0+e],[0 0 1 1-e 0+e 0+e],c2);patch([0 0 1 1-e 0+e 0+e],[0 1 1 1-e 1-e 0+e],c3);plot([0 1 1 0 0],[0 0 1 1 0]);disp('weights');
  Mux : Mux  Inputs=10
      mask Display: e = 0.06;c1 = [120 150 230]/255;c2 = ([120 150 230]+0)/383;c3 = ([120 150 230]+128)/383;patch([0 1 1 0],[0 0 1 1],c1);patch([0 1 1 1-e 1-e 0+e],[0 0 1 1-e 0+e 0+e],c2);patch([0 0 1 1-e 0+e 0+e],[0 1 1 1-e 1-e 0+e],c3);plot([0 1 1 0 0],[0 0 1 1 0]);disp('Mux');
  dotprod{1..10} (10 alike) : neural/Weight Functions/dotprod
  "lz{2,1}" : Outport
      mask Display: e = 0.06;c1 = [120 230 180]/255;c2 = ([120 230 180]+0)/(256+128);c3 = ([120 230 180]+128)/(256+128);patch([0 1 1 0],[0 0 1 1],c1);patch([0 1 1 1-e 1-e 0+e],[0 0 1 1-e 0+e 0+e],c2);patch([0 0 1 1-e 0+e 0+e],[0 1 1 1-e 1-e 0+e],c3);plot([0 1 1 0 0],[0 0 1 1 0]);
  wires:
  Mux/1 -> "lz{2,1}"/1
  dotprod10/1 -> Mux/10
  "IW{2,1}(10,:)'"/1 -> dotprod10/1
  dotprod9/1 -> Mux/9
  "IW{2,1}(9,:)'"/1 -> dotprod9/1
  dotprod8/1 -> Mux/8
  "IW{2,1}(8,:)'"/1 -> dotprod8/1
  dotprod7/1 -> Mux/7
  "IW{2,1}(7,:)'"/1 -> dotprod7/1
  dotprod6/1 -> Mux/6
  "IW{2,1}(6,:)'"/1 -> dotprod6/1
  dotprod5/1 -> Mux/5
  "IW{2,1}(5,:)'"/1 -> dotprod5/1
  dotprod4/1 -> Mux/4
  "IW{2,1}(4,:)'"/1 -> dotprod4/1
  dotprod3/1 -> Mux/3
  "IW{2,1}(3,:)'"/1 -> dotprod3/1
  dotprod2/1 -> Mux/2
  "IW{2,1}(2,:)'"/1 -> dotprod2/1
  dotprod1/1 -> Mux/1
  "ad{2,1}"/1 -> dotprod10/2, dotprod9/2, dotprod8/2, dotprod7/2, dotprod6/2, dotprod5/2, dotprod4/2, dotprod3/2, dotprod2/2, dotprod1/2
  "IW{2,1}(1,:)'"/1 -> dotprod1/1

== system Lcontainer_simNN/LContainer Plant/Layer 3/Delays 1 ==
  "p{3}" : Inport  PortDimensions=10
      mask Display: e = 0.06;c1 = [120 230 180]/255;c2 = ([120 230 180]+0)/(256+128);c3 = ([120 230 180]+128)/(256+128);patch([0 1 1 0],[0 0 1 1],c1);patch([0 1 1 1-e 1-e 0+e],[0 0 1 1-e 0+e 0+e],c2);patch([0 0 1 1-e 0+e 0+e],[0 1 1 1-e 1-e 0+e],c3);plot([0 1 1 0 0],[0 0 1 1 0]);
  mux : Mux  Inputs=1
      mask Display: e = 0.06;c1 = [120 150 230]/255;c2 = ([120 150 230]+0)/383;c3 = ([120 150 230]+128)/383;patch([0 1 1 0],[0 0 1 1],c1);patch([0 1 1 1-e 1-e 0+e],[0 0 1 1-e 0+e 0+e],c2);patch([0 0 1 1-e 0+e 0+e],[0 1 1 1-e 1-e 0+e],c3);plot([0 1 1 0 0],[0 0 1 1 0]);disp('Mux')
  "pd{3,2}" : Outport
      mask Display: e = 0.06;c1 = [120 230 180]/255;c2 = ([120 230 180]+0)/(256+128);c3 = ([120 230 180]+128)/(256+128);patch([0 1 1 0],[0 0 1 1],c1);patch([0 1 1 1-e 1-e 0+e],[0 0 1 1-e 0+e 0+e],c2);patch([0 0 1 1-e 0+e 0+e],[0 1 1 1-e 1-e 0+e],c3);plot([0 1 1 0 0],[0 0 1 1 0]);
  wires:
  mux/1 -> "pd{3,2}"/1
  "p{3}"/1 -> mux/1
